simulink model "model"  (R2020b)
settings: Solver=ode15s  StartTime=0.0  StopTime=data.detumbling.times(end)  MaxStep=0.2  RelTol=1e-8  AbsTol=1e-8
libraries: libraryMatlab x4
settings Model: Creator=pacif  LastModifiedBy=pacif

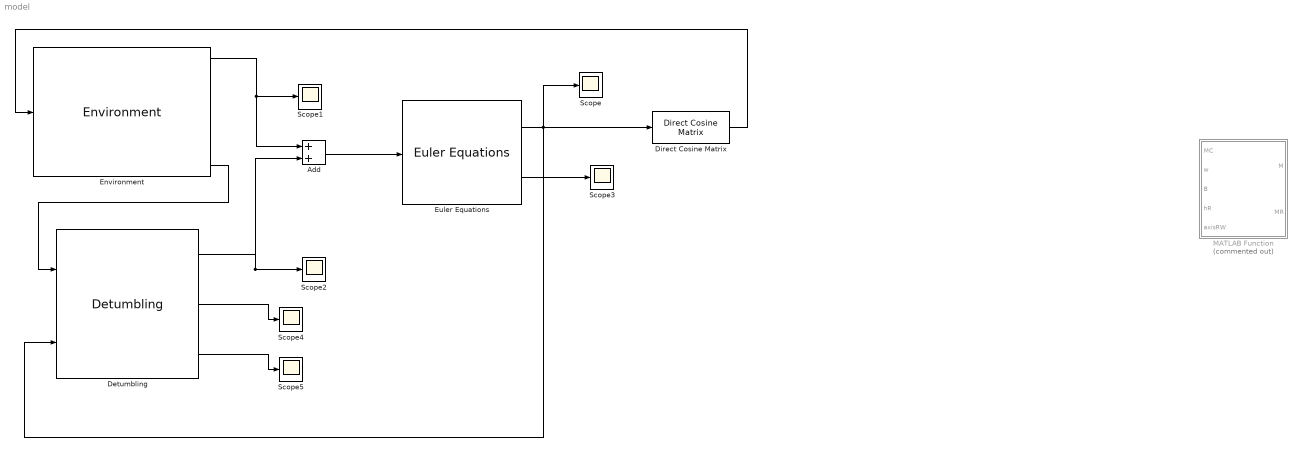
== system model ==
  Add : Sum
  Detumbling : libraryMatlab/Detumbling  SystemSampleTime=-1  VariantActivationTime=update diagram  Latency=0  AutoFrameSizeCalculation=off
  Direct Cosine Matrix : libraryMatlab/Direct Cosine Matrix  SystemSampleTime=-1  VariantActivationTime=update diagram  Latency=0  AutoFrameSizeCalculation=off
  Environment : libraryMatlab/Environment  SystemSampleTime=-1  VariantActivationTime=update diagram  Latency=0  AutoFrameSizeCalculation=off
  Euler Equations : libraryMatlab/Euler Equations  SystemSampleTime=-1  VariantActivationTime=update diagram  Latency=0  AutoFrameSizeCalculation=off
  MATLAB Function : MATLAB Function  Commented=on  TreatAsAtomicUnit=on
  Scope{,1..5} (6 alike) : Scope
  wires:
  Euler Equations/1 -> Detumbling/2, Direct Cosine Matrix/1, Scope/1
  Direct Cosine Matrix/1 -> Environment/1
  Add/1 -> Euler Equations/1
  Environment/1 -> Scope1/1, Add/1
  Detumbling/1 -> Add/2, Scope2/1
  Environment/5 -> Detumbling/1
  Euler Equations/2 -> Scope3/1
  Detumbling/2 -> Scope4/1
  Detumbling/3 -> Scope5/1

== matlab function model/MATLAB Function ==
  data: MC input; M output; w input; B input; hR input; axisRW input; MR output
function [M,MR] = fun(MC, w, B, hR, axisRW)

MC1 = MC + cross(w,hR*axisRW);

Bx = B(1); By = B(2); Bz = B(3);

% C = [0      Bz      -By     0
%     -Bz     0       Bx      0
%     By      -Bx     0       -1];
% 
% invC = pinv(C);
% 
% u = invC*MC1;
% 
% D = u(1:3)*normB; MR = u(4);
% 
% if abs(D(1)) > 140, D(1) = sign(D(1))*140; end
% if abs(D(2)) > 140, D(2) = sign(D(2))*140; end

Dx = -MC1(2)/Bz; Dy = MC1(1)/Bz;

if abs(Dx) > 140, Dx = sign(Dx)*140; end
if abs(Dy) > 140, Dy = sign(Dy)*140; end

MR = -MC1(3) + By*Dx - Bx*Dy;

if abs(MR) > 18; MR = sign(MR)*18; end
% % if hR >= 0.2 && MR > 0, MR = 0; end
% % if hR <= -0.2 && MR < 0, MR = 0; end

D = [Dx; Dy; 0]; 

M1 = cross(D,B);

M2 = -cross(w,axisRW*hR) - axisRW*MR;


M = M1 + M2;

    


end
